simulink model "dosestres"  (R2012b)
settings: Solver=ode45  StartTime=0.0  StopTime=10.0  RelTol=1e-3
undefined symbols (not defined in the file or in its folder): dostres
libraries: simulink x2
settings Model: Creator=Daniel  LastModifiedBy=Daniel

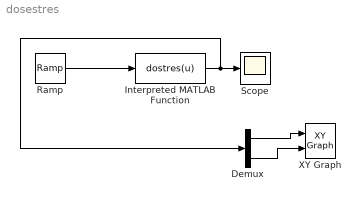
== system dosestres ==
  Demux : Demux  Outputs=2
  Interpreted MATLAB Function : MATLABFcn  MATLABFcn=dostres(u)  OutputDimensions=2
  Ramp : simulink/Sources/Ramp  slope=1  start=0  X0=0
  Scope : Scope
  XY Graph : simulink/Sinks/XY Graph  xmin=-1  xmax=1  ymin=-1  ymax=1  st=-1
  wires:
  Ramp/1 -> Interpreted MATLAB Function/1
  Interpreted MATLAB Function/1 -> Demux/1, Scope/1
  Demux/1 -> XY Graph/1
  Demux/2 -> XY Graph/2
